simulink library "Lib_MCHP_BLKDEMO_Motor"  (R2015b)
settings: Solver=VariableStepAuto  StartTime=0.0  StopTime=10.0  RelTol=1e-3
values from neighbouring files (symbols this model uses):
  DEADTIME = 1e-6    (= 1e-06)    [UserParams.m]
  PSHIFT = TConv/2    (= 4.680375e-06)    [UserParams.m]
  PWMFREQUENCY = 20e3    (= 20000)    [UserParams.m]
  TSETTLE = 2e-6    (= 2e-06)    [UserParams.m]
  TSmp = 0.343*1e-6    (= 3.43e-07)    [UserParams.m]
undefined symbols (not defined in the file or in its folder): A4, B15, B9, C6, F0, P20, P41, P47, P54, P96, Pin, PWMmax, XData
libraries: MCHP_Blockset x9, simulink x7, Lib_MCHP_BLKDEMO_Motor x6
(part 2 of 2)

== system Lib_MCHP_BLKDEMO_Motor/MOTOR/SINGLE SHUNT Edge Aligned/MOTOR - Board Sensor/encoder scaled ==
  Rst : Inport
  Direct Lookup Table (n-D) : LookupNDDirect  NumberOfTableDimensions=1  Table=[0:199]*inv(200)  TableDataTypeStr=fixdt(0,16,16)
      settings: LockScale=on
  Q0.4 : DataTypeConversion
  QEI : MCHP_Blockset/QEI/QEI  QEI_REF=1  QEI_MODE=Quadrature Encoder  QEI_x2mode=off  QEI_PulseCountDir=Down  PIN_QEA=Dynamic Options  PIN_QEA_TXT=C6 / P54 / Pin[50]  PIN_QEB=Dynamic Options  PIN_QEB_TXT=F0 / P96 / Pin[58]  SWPAB=on  QEAPOL=off  QEBPOL=off  SampleTime=-1  INDXxCNT_Output=is not an output  POSxCNT_Output=is a 16 bits unsigned block output  RESET_Input=on  PIMOD_mode=position is cyclique between user defined boundaries  PIMOD_modeB=Never reset position  PIMOD_reset=on next INDEX event  PIN_INDEX=Dynamic Options  PIN_INDEX_TXT=B15 / P47 / Pin[3]  IMV=QEA = 1 and QEB = 0  IMV_x2=QEA = 1  PIN_HOME=Dynamic Options  PIN_HOME_TXT=B9 / P41 / Pin[49]  QEIxLEC_GEC=[0 199]  QEIxIC=0  PCIIRQ=off  IDXPOL=off  HOMPOL=on  VELxCNT_Output=is not an output  INTxHLD_Output=is not an output  MaxPeriod=0.1  FILTREN=on  QFDIV_popup=Dynamic Options  QFDIV_popup_TXT=364.58 kHz  FILTER_CutOffFreq=100e3  PIN_CCMP=Dynamic Options  PIN_CCMP_TXT=A4 / P20 / Pin[33]  MCHP_PORT={QEI1 A}{QEA1}5:0:P54;{QEI1 B}{QEB1}5:0:P96;  MCHP_MASTERLINK=Test_PWMHS_33EP256MC506/Microchip Master  QEI_IntPri=5
  Rate Transition4 : RateTransition  X0=1
  theta_enc_fract : Outport
  wires:
  Rate Transition4/1 -> QEI/1
  Q0.4/1 -> Rate Transition4/1
  Rst/1 -> Q0.4/1
  Direct Lookup Table (n-D)/1 -> theta_enc_fract/1
  QEI/1 -> Direct Lookup Table (n-D)/1

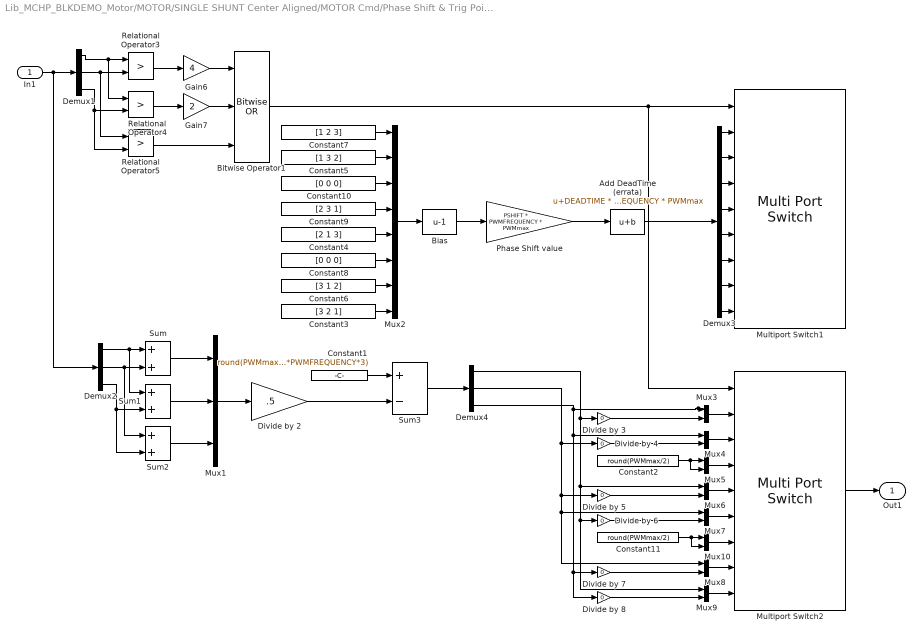
== system Lib_MCHP_BLKDEMO_Motor/MOTOR/SINGLE SHUNT Center Aligned/MOTOR Cmd/Phase Shift & Trig Point/Phase Shift1 ==
  In1 : Inport
  Add DeadTime (errata) : Bias  Bias=DEADTIME * PWMFREQUENCY * PWMmax  SaturateOnIntegerOverflow=on
  Bias : Bias  Bias=-1  SaturateOnIntegerOverflow=on
  Bitwise Operator1 : simulink/Logic and Bit Operations/Bitwise Operator  logicop=OR  UseBitMask=off  NumInputPorts=3  BitMask=bin2dec('11011001')  BitMaskRealWorld=Stored Integer
  Constant1 : Constant  Value=round(PWMmax + DEADTIME*PWMmax*PWMFREQUENCY*3)  OutDataTypeStr=Inherit: Inherit via back propagation
  Constant10 : Constant  Value=[0 0 0]  OutDataTypeStr=int16
  Constant11 : Constant  Value=round(PWMmax/2)  OutDataTypeStr=Inherit: Inherit via back propagation
  Constant2 : Constant  Value=round(PWMmax/2)  OutDataTypeStr=Inherit: Inherit via back propagation
  Constant3 : Constant  Value=[3 2 1]  OutDataTypeStr=int16
  Constant4 : Constant  Value=[2 1 3]  OutDataTypeStr=int16
  Constant5 : Constant  Value=[1 3 2]  OutDataTypeStr=int16
  Constant6 : Constant  Value=[3 1 2]  OutDataTypeStr=int16
  Constant7 : Constant  Value=[1 2 3]  OutDataTypeStr=int16
  Constant8 : Constant  Value=[0 0 0]  OutDataTypeStr=int16
  Constant9 : Constant  Value=[2 3 1]  OutDataTypeStr=int16
  Demux1 : Demux  Outputs=3
  Demux2 : Demux  Outputs=3
  Demux3 : Demux  Outputs=8
  Demux4 : Demux  Outputs=3
  Divide by 2 : Gain  Gain=.5  SaturateOnIntegerOverflow=on  OutDataTypeStr=Inherit: Same as input
  Divide by {3..8} (6 alike) : Gain  Gain=0  SaturateOnIntegerOverflow=on  OutDataTypeStr=Inherit: Same as input
  Gain6 : Gain  Gain=4  OutDataTypeStr=Inherit: Same as input
  Gain7 : Gain  Gain=2  OutDataTypeStr=Inherit: Same as input
  Multiport Switch1 : MultiPortSwitch  DataPortOrder=Zero-based contiguous  Inputs=8  DiagnosticForDefault=None
  Multiport Switch2 : MultiPortSwitch  DataPortOrder=Zero-based contiguous  Inputs=8  DiagnosticForDefault=None
  Mux1 : Mux  Inputs=3
  Mux{3..10} (8 alike) : Mux  Inputs=2
  Mux2 : Mux  Inputs=8
  Phase Shift value : Gain  Gain=PSHIFT * PWMFREQUENCY * PWMmax  OutDataTypeStr=uint16  SaturateOnIntegerOverflow=on
  Relational Operator3 : RelationalOperator  Operator=>  OutDataTypeStr=fixdt(1,16)
  Relational Operator4 : RelationalOperator  Operator=>  OutDataTypeStr=fixdt(1,16)
  Relational Operator5 : RelationalOperator  Operator=>  OutDataTypeStr=fixdt(1,16)
  Sum : Sum
  Sum1 : Sum
  Sum2 : Sum
  Sum3 : Sum  Inputs=+-  OutDataTypeStr=Inherit: Inherit via back propagation
  Out1 : Outport
  wires:
  Divide by 7/1 -> Mux8/2
  Divide by 8/1 -> Mux9/2
  Divide by 6/1 -> Mux7/2
  Divide by 5/1 -> Mux6/2
  Divide by 4/1 -> Mux4/2
  Divide by 3/1 -> Mux3/2
  Demux4/3 -> Mux4/1, Divide by 8/1, Divide by 7/1, Mux3/1
  Sum3/1 -> Demux4/1
  Multiport Switch2/1 -> Out1/1
  Constant11/1 -> Mux10/1, Mux10/2
  Constant2/1 -> Mux5/1, Mux5/2
  Mux10/1 -> Multiport Switch2/7
  Mux9/1 -> Multiport Switch2/9
  Mux8/1 -> Multiport Switch2/8
  Mux7/1 -> Multiport Switch2/6
  Mux6/1 -> Multiport Switch2/5
  Mux5/1 -> Multiport Switch2/4
  Demux4/2 -> Divide by 4/1, Mux8/1, Mux7/1, Divide by 5/1
  Mux4/1 -> Multiport Switch2/3
  Demux4/1 -> Divide by 3/1, Divide by 6/1, Mux9/1, Mux6/1
  Mux3/1 -> Multiport Switch2/2
  Constant1/1 -> Sum3/1
  Divide by 2/1 -> Sum3/2
  Mux1/1 -> Divide by 2/1
  Sum2/1 -> Mux1/3
  Sum1/1 -> Mux1/2
  Sum/1 -> Mux1/1
  Demux2/3 -> Sum1/2, Sum2/2
  Demux2/2 -> Sum/2, Sum2/1
  Demux2/1 -> Sum/1, Sum1/1
  Add DeadTime (errata)/1 -> Demux3/1
  Bias/1 -> Phase Shift value/1
  Constant3/1 -> Mux2/8
  Constant6/1 -> Mux2/7
  Constant8/1 -> Mux2/6
  Constant4/1 -> Mux2/5
  Constant9/1 -> Mux2/4
  Constant10/1 -> Mux2/3
  Constant5/1 -> Mux2/2
  Constant7/1 -> Mux2/1
  Demux1/1 -> Relational Operator3/1, Relational Operator4/1
  Relational Operator4/1 -> Gain7/1
  Demux1/3 -> Relational Operator4/2, Relational Operator5/2
  In1/1 -> Demux1/1, Demux2/1
  Demux1/2 -> Relational Operator3/2, Relational Operator5/1
  Relational Operator3/1 -> Gain6/1
  Demux3/6 -> Multiport Switch1/7
  Phase Shift value/1 -> Add DeadTime (errata)/1
  Demux3/1 -> Multiport Switch1/2
  Relational Operator5/1 -> Bitwise Operator1/3
  Mux2/1 -> Bias/1
  Demux3/4 -> Multiport Switch1/5
  Demux3/7 -> Multiport Switch1/8
  Demux3/3 -> Multiport Switch1/4
  Demux3/5 -> Multiport Switch1/6
  Gain6/1 -> Bitwise Operator1/1
  Demux3/8 -> Multiport Switch1/9
  Demux3/2 -> Multiport Switch1/3
  Gain7/1 -> Bitwise Operator1/2
  Bitwise Operator1/1 -> Multiport Switch1/1, Multiport Switch2/1

== system Lib_MCHP_BLKDEMO_Motor/MOTOR/SINGLE SHUNT Center Aligned/MOTOR Cmd/Phase Shift & Trig Point/Subsystem1 ==
  In : Inport
  Bias : Inport  Port=2
  Sum7 : Sum  Inputs=|++  OutDataTypeStr=Inherit: Same as accumulator
  Sum8 : Sum  Inputs=|+-  OutDataTypeStr=Inherit: Same as accumulator
  Out bias+ : Outport
  Out bias- : Outport  Port=2
  wires:
  Sum8/1 -> Out bias-/1
  Sum7/1 -> Out bias+/1
  In/1 -> Sum7/1, Sum8/1
  Bias/1 -> Sum7/2, Sum8/2

== system Lib_MCHP_BLKDEMO_Motor/MOTOR/SINGLE SHUNT Center Aligned/MOTOR Cmd/Phase Shift & Trig Point/Subsystem10 ==
  In : Inport
  Bias : Inport  Port=2
  Sum7 : Sum  Inputs=|++  OutDataTypeStr=Inherit: Same as accumulator
  Sum8 : Sum  Inputs=|+-  OutDataTypeStr=Inherit: Same as accumulator
  Out bias+ : Outport
  Out bias- : Outport  Port=2
  wires:
  Bias/1 -> Sum8/2, Sum7/2
  In/1 -> Sum8/1, Sum7/1
  Sum7/1 -> Out bias+/1
  Sum8/1 -> Out bias-/1

== system Lib_MCHP_BLKDEMO_Motor/MOTOR/SINGLE SHUNT Center Aligned/MOTOR Cmd/Phase Shift & Trig Point/Subsystem11 ==
  In : Inport
  Bias : Inport  Port=2
  Sum7 : Sum  Inputs=|++  OutDataTypeStr=Inherit: Same as accumulator
  Sum8 : Sum  Inputs=|+-  OutDataTypeStr=Inherit: Same as accumulator
  Out bias+ : Outport
  Out bias- : Outport  Port=2
  wires:
  Sum8/1 -> Out bias-/1
  Sum7/1 -> Out bias+/1
  In/1 -> Sum7/1, Sum8/1
  Bias/1 -> Sum7/2, Sum8/2

== system Lib_MCHP_BLKDEMO_Motor/MOTOR/SINGLE SHUNT Center Aligned/MOTOR Cmd/Phase Shift & Trig Point/Subsystem12 ==
  In : Inport
  Bias : Inport  Port=2
  Sum7 : Sum  Inputs=|++  OutDataTypeStr=Inherit: Same as accumulator
  Sum8 : Sum  Inputs=|+-  OutDataTypeStr=Inherit: Same as accumulator
  Out bias+ : Outport
  Out bias- : Outport  Port=2
  wires:
  Bias/1 -> Sum8/2, Sum7/2
  In/1 -> Sum8/1, Sum7/1
  Sum7/1 -> Out bias+/1
  Sum8/1 -> Out bias-/1

== system Lib_MCHP_BLKDEMO_Motor/MOTOR/SINGLE SHUNT Center Aligned/MOTOR Cmd/Phase Shift & Trig Point/Subsystem2 ==
  In : Inport
  Bias : Inport  Port=2
  Sum7 : Sum  Inputs=|++  OutDataTypeStr=Inherit: Same as accumulator
  Sum8 : Sum  Inputs=|+-  OutDataTypeStr=Inherit: Same as accumulator
  Out bias+ : Outport
  Out bias- : Outport  Port=2
  wires:
  Bias/1 -> Sum8/2, Sum7/2
  In/1 -> Sum8/1, Sum7/1
  Sum7/1 -> Out bias+/1
  Sum8/1 -> Out bias-/1

== system Lib_MCHP_BLKDEMO_Motor/MOTOR/SINGLE SHUNT Center Aligned/MOTOR Cmd/Phase Shift & Trig Point/Subsystem3 ==
  In : Inport
  Bias : Inport  Port=2
  Sum7 : Sum  Inputs=|++  OutDataTypeStr=Inherit: Same as accumulator
  Sum8 : Sum  Inputs=|+-  OutDataTypeStr=Inherit: Same as accumulator
  Out bias+ : Outport
  Out bias- : Outport  Port=2
  wires:
  Bias/1 -> Sum8/2, Sum7/2
  In/1 -> Sum8/1, Sum7/1
  Sum7/1 -> Out bias+/1
  Sum8/1 -> Out bias-/1

== system Lib_MCHP_BLKDEMO_Motor/MOTOR/SINGLE SHUNT Center Aligned/MOTOR Cmd/Phase Shift & Trig Point/Subsystem4 ==
  In : Inport
  Bias : Inport  Port=2
  Sum7 : Sum  Inputs=|++  OutDataTypeStr=Inherit: Same as accumulator
  Sum8 : Sum  Inputs=|+-  OutDataTypeStr=Inherit: Same as accumulator
  Out bias+ : Outport
  Out bias- : Outport  Port=2
  wires:
  Sum8/1 -> Out bias-/1
  Sum7/1 -> Out bias+/1
  In/1 -> Sum7/1, Sum8/1
  Bias/1 -> Sum7/2, Sum8/2

== system Lib_MCHP_BLKDEMO_Motor/MOTOR/SINGLE SHUNT Center Aligned/MOTOR Cmd/Phase Shift & Trig Point/Subsystem5 ==
  In : Inport
  Bias : Inport  Port=2
  Sum7 : Sum  Inputs=|++  OutDataTypeStr=Inherit: Same as accumulator
  Sum8 : Sum  Inputs=|+-  OutDataTypeStr=Inherit: Same as accumulator
  Out bias+ : Outport
  Out bias- : Outport  Port=2
  wires:
  Sum8/1 -> Out bias-/1
  Sum7/1 -> Out bias+/1
  In/1 -> Sum7/1, Sum8/1
  Bias/1 -> Sum7/2, Sum8/2

== system Lib_MCHP_BLKDEMO_Motor/MOTOR/SINGLE SHUNT Center Aligned/MOTOR Cmd/Phase Shift & Trig Point/Subsystem6 ==
  In : Inport
  Bias : Inport  Port=2
  Sum7 : Sum  Inputs=|++  OutDataTypeStr=Inherit: Same as accumulator
  Sum8 : Sum  Inputs=|+-  OutDataTypeStr=Inherit: Same as accumulator
  Out bias+ : Outport
  Out bias- : Outport  Port=2
  wires:
  Bias/1 -> Sum8/2, Sum7/2
  In/1 -> Sum8/1, Sum7/1
  Sum7/1 -> Out bias+/1
  Sum8/1 -> Out bias-/1

== system Lib_MCHP_BLKDEMO_Motor/MOTOR/SINGLE SHUNT Center Aligned/MOTOR Cmd/Phase Shift & Trig Point/Subsystem7 ==
  In : Inport
  Bias : Inport  Port=2
  Sum7 : Sum  Inputs=|++  OutDataTypeStr=Inherit: Same as accumulator
  Sum8 : Sum  Inputs=|+-  OutDataTypeStr=Inherit: Same as accumulator
  Out bias+ : Outport
  Out bias- : Outport  Port=2
  wires:
  Bias/1 -> Sum8/2, Sum7/2
  In/1 -> Sum8/1, Sum7/1
  Sum7/1 -> Out bias+/1
  Sum8/1 -> Out bias-/1

== system Lib_MCHP_BLKDEMO_Motor/MOTOR/SINGLE SHUNT Center Aligned/MOTOR Cmd/Phase Shift & Trig Point/Subsystem8 ==
  In : Inport
  Bias : Inport  Port=2
  Sum7 : Sum  Inputs=|++  OutDataTypeStr=Inherit: Same as accumulator
  Sum8 : Sum  Inputs=|+-  OutDataTypeStr=Inherit: Same as accumulator
  Out bias+ : Outport
  Out bias- : Outport  Port=2
  wires:
  Sum8/1 -> Out bias-/1
  Sum7/1 -> Out bias+/1
  In/1 -> Sum7/1, Sum8/1
  Bias/1 -> Sum7/2, Sum8/2

== system Lib_MCHP_BLKDEMO_Motor/MOTOR/SINGLE SHUNT Center Aligned/MOTOR Cmd/Phase Shift & Trig Point/Subsystem9 ==
  In : Inport
  Bias : Inport  Port=2
  Sum7 : Sum  Inputs=|++  OutDataTypeStr=Inherit: Same as accumulator
  Sum8 : Sum  Inputs=|+-  OutDataTypeStr=Inherit: Same as accumulator
  Out bias+ : Outport
  Out bias- : Outport  Port=2
  wires:
  Sum8/1 -> Out bias-/1
  Sum7/1 -> Out bias+/1
  In/1 -> Sum7/1, Sum8/1
  Bias/1 -> Sum7/2, Sum8/2
